simulink model "s_lqr3"  (Simulink 4.00)
settings: Solver=ode45  SolverMode=SingleTasking  StartTime=0.0  StopTime=200  MaxStep=0.10  RelTol=1e-3  AbsTol=1e-6
values from neighbouring files (symbols this model uses):
  C = [Cp, zeros(1,ns)]    [akalm1.m]    (also in kalm1.m = my_sys1.c; kalm2.m = my_sys1.c; kalm3.m = my_sys1.c; kalm4.m = [eye(3,3), zeros(3,3)])
  k6 = K(n)    [lqr_1.m]    (also in lqr_2.m; lqr_3.m)
  x0 = [5, 0, 0, 0]    [abeob1.m]    (also in alqr1.m; alqrd1.m; apol1.m; estimate_1.m = [1 2 3])
settings Model: LastModifiedBy=Administrator  SaveTime=off  SaveOutput=off  LimitDataPoints=off  BlockReductionOpt=off

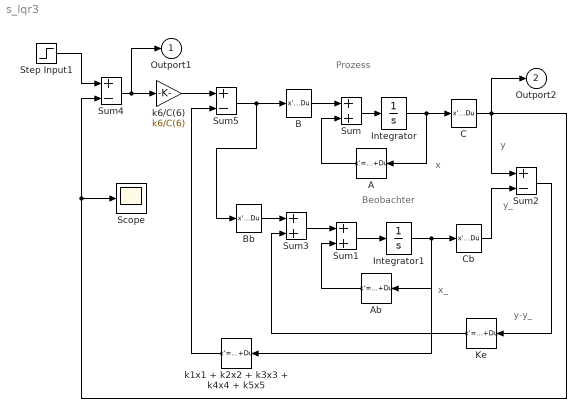
== system s_lqr3 ==
  note: Prozess
  note: y
  note: x
  note: x_
  note: Beobachter
  note: y_
  note: y-y_
  A : StateSpace  Orientation=left  A=[]  B=[]  C=[]  D=K  X0=0  Realization=auto  AbsoluteTolerance=auto  mask(Matrix Gain){@1=A}
      mask prompts: @1 "Gain matrix:"
      mask help: Matrix Gain.
      mask init:
      | K = @1;
      mask Help: Multiplies input vector by entered matrix to produce output vector (y=Au).
      mask Display: disp('K')
  Ab : StateSpace  Orientation=left  A=[]  B=[]  C=[]  D=K  X0=0  Realization=auto  AbsoluteTolerance=auto  mask(Matrix Gain){@1=Ab}
      mask prompts: @1 "Gain matrix:"
      mask help: Matrix Gain.
      mask init:
      | K = @1;
      mask Help: Multiplies input vector by entered matrix to produce output vector (y=Au).
      mask Display: disp('K')
  B : StateSpace  A=[]  B=[]  C=[]  D=K  X0=0  Realization=auto  AbsoluteTolerance=auto  mask(Matrix Gain){@1=B}
      mask prompts: @1 "Gain matrix:"
      mask help: Matrix Gain.
      mask init:
      | K = @1;
      mask Help: Multiplies input vector by entered matrix to produce output vector (y=Au).
      mask Display: disp('K')
  Bb : StateSpace  A=[]  B=[]  C=[]  D=K  X0=0  Realization=auto  AbsoluteTolerance=auto  mask(Matrix Gain){@1=Bb}
      mask prompts: @1 "Gain matrix:"
      mask help: Matrix Gain.
      mask init:
      | K = @1;
      mask Help: Multiplies input vector by entered matrix to produce output vector (y=Au).
      mask Display: disp('K')
  C : StateSpace  A=[]  B=[]  C=[]  D=K  X0=0  Realization=auto  AbsoluteTolerance=auto  mask(Matrix Gain){@1=C}
      mask prompts: @1 "Gain matrix:"
      mask help: Matrix Gain.
      mask init:
      | K = @1;
      mask Help: Multiplies input vector by entered matrix to produce output vector (y=Au).
      mask Display: disp('K')
  Cb : StateSpace  A=[]  B=[]  C=[]  D=K  X0=0  Realization=auto  AbsoluteTolerance=auto  mask(Matrix Gain){@1=Cb}
      mask prompts: @1 "Gain matrix:"
      mask help: Matrix Gain.
      mask init:
      | K = @1;
      mask Help: Multiplies input vector by entered matrix to produce output vector (y=Au).
      mask Display: disp('K')
  Integrator : Integrator  ExternalReset=none  InitialConditionSource=internal  InitialCondition=[x0]  LimitOutput=off  UpperSaturationLimit=inf  LowerSaturationLimit=-inf  ShowSaturationPort=off  ShowStatePort=off  AbsoluteTolerance=auto
  Integrator1 : Integrator  ExternalReset=none  InitialConditionSource=internal  InitialCondition=[0]  LimitOutput=off  UpperSaturationLimit=inf  LowerSaturationLimit=-inf  ShowSaturationPort=off  ShowStatePort=off  AbsoluteTolerance=auto
  Ke : StateSpace  Orientation=left  A=[]  B=[]  C=[]  D=K  X0=0  Realization=auto  AbsoluteTolerance=auto  mask(Matrix Gain){@1=Ke}
      mask prompts: @1 "Gain matrix:"
      mask help: Matrix Gain.
      mask init:
      | K = @1;
      mask Help: Multiplies input vector by entered matrix to produce output vector (y=Au).
      mask Display: disp('K')
  Scope : Scope
      settings: TickLabels=on  TimeRange=200.000000  YMin=-10.600000  YMax=10.600000  SaveToWorkspace=off  SaveName=ScopeData  DataFormat=Array  LimitDataPoints=on  MaxDataPoints=5000
  Step Input1 : Step  Time=0  Before=0  After=1  SampleTime=0
  Sum : Sum  Inputs=++  SaturateOnIntegerOverflow=on
  Sum1 : Sum  Inputs=++  SaturateOnIntegerOverflow=on
  Sum2 : Sum  Inputs=+-  SaturateOnIntegerOverflow=on
  Sum3 : Sum  Inputs=++  SaturateOnIntegerOverflow=on
  Sum4 : Sum  Inputs=+-  SaturateOnIntegerOverflow=on
  Sum5 : Sum  Inputs=+-  SaturateOnIntegerOverflow=on
  k1x1 + k2x2 + k3x3 + k4x4 + k5x5 : StateSpace  Orientation=left  A=[]  B=[]  C=[]  D=K  X0=0  Realization=auto  AbsoluteTolerance=auto  mask(Matrix Gain){@1=k15}
      mask prompts: @1 "Gain matrix:"
      mask help: Matrix Gain.
      mask init:
      | K = @1;
      mask Help: Multiplies input vector by entered matrix to produce output vector (y=Au).
      mask Display: disp('K')
  k6/C(6) : Gain  Gain=k6/C(6)  Multiplication=Element-wise(K.*u)  SaturateOnIntegerOverflow=on
  Outport1 : Outport  Port=1  InitialOutput=0
  Outport2 : Outport  Port=2  InitialOutput=0
  wires:
  Integrator1/1 -> k1x1 + k2x2 + k3x3 + k4x4 + k5x5/1, Cb/1, Ab/1
  k1x1 + k2x2 + k3x3 + k4x4 + k5x5/1 -> Sum5/2
  Sum5/1 -> Bb/1, B/1
  k6/C(6)/1 -> Sum5/1
  Sum4/1 -> Outport1/1, k6/C(6)/1
  C/1 -> Scope/1, Sum4/2, Outport2/1, Sum2/1
  Step Input1/1 -> Sum4/1
  Bb/1 -> Sum3/1
  Ke/1 -> Sum3/2
  Sum2/1 -> Ke/1
  Sum3/1 -> Sum1/1
  Cb/1 -> Sum2/2
  Ab/1 -> Sum1/2
  Sum1/1 -> Integrator1/1
  Integrator/1 -> C/1, A/1
  A/1 -> Sum/2
  Sum/1 -> Integrator/1
  B/1 -> Sum/1
